simulink model "MMADC"  (R2021a)
settings: Solver=VariableStepAuto  StartTime=0.0  StopTime=1  RelTol=1e-3
values from neighbouring files (symbols this model uses):
  Cf = minimum_cap    [MMADC_main.m]
  clk_freq = 2.1*(nb_MAC+1)/nb_MAC*input_BW    (= 1684.375)    [MMADC_main.m]
  clk_period = 1/clk_freq    (= 0.000593692022263)    [MMADC_main.m]
  comparator_high_offset = 0.2*10e-4    (= 0.0002)    [MMADC_main.m]
  comparator_low_offset = -.1*10e-4    (= -0.0001)    [MMADC_main.m]
  comparator_noise_on = noise_on    (= 1)    [MMADC_main.m]
  comparator_noise_rms = 1*k*T* 2/3 / minimum_cap    [MMADC_main.m]
  comparator_offset_on = noise_on    (= 1)    [MMADC_main.m]
  k = 1.38064852e-23    [MMADC_main.m]
  LNA_bandwidth = 2.5*input_BW    (= 2000)    [MMADC_main.m]
  LNA_gain = 10^(36/20)*12*1.5849    (= 1200.00515432)    [MMADC_main.m]
  LNA_input_referred_noise = sqrt(pi/2*LNA_bandwidth*(194*10^-9)^2)    [MMADC_main.m]
  LNA_noise_on = noise_on    (= 1)    [MMADC_main.m]
  MM_incomplete_transfer_coeff = C1/(C1+C2)    [MMADC_main.m]
  MM_leakage_per_clk_cycle = 1    [MMADC_main.m]
  MM_sampling_noise = noise_on*((k*T * C1/(C1+C2)^2) + (k*T*(C1*C2/(C1+C2))/C2^2))    [MMADC_main.m]
  nb_MAC = 384    [MMADC_main.m]
  number_of_bits = 6    [MMADC_main.m]
  sample_time_jitter = 16e-12    (= 1.6e-11)    [MMADC_main.m]
  sampling_gain = Cs/Cf    [MMADC_main.m]
  sampling_jitter_on = noise_on    (= 1)    [MMADC_main.m]
  sensing_matrix = sensing_matrix_large(j:j+min(19,i-1),:)    [MMADC_main.m]
  sim_number = 0    [MMADC_main.m]
  switch_noise_on = noise_on    (= 1)    [MMADC_main.m]
  switching_noise = k*T/Cf    [MMADC_main.m]
  T = 293    [MMADC_main.m]
  Vref = 2    [MMADC_main.m]
  ZOH_delta = 0*Vref/(2^number_of_bits)    (= 0)    [MMADC_main.m]
libraries: simulink x100, simulink_extras x41, dspsigops x21, dspsrcs4 x21, spsFirstOrderFilterLib x1, dspswit3 x1
(part 2 of 10)

== system MMADC/Sensing Channel 8 ==
  In5 : Inport
  Input : Inport  Port=2
  AND : Logic  IconShape=distinctive  AllPortsSameDT=off  OutDataTypeStr=boolean
  Bus Selector : BusSelector  OutputSignals=reset MAC,trigger MAC,sample SAR,trigger SAR
  SAR : Subsystem
      mask Display: text(.5, .5, 'ZOH SAR', 'horizontalAlignment', 'center', 'verticalAlignment', 'middle')
  Sample&hold : Subsystem
      settings: PortSchema="{\"entries\":[{\"content\":{\"sides\":[{\"content\":{\"connectorIds\":[\"In1\"]},\"type\":\"ConnectorPlacement.EquallySpacedRectSide\",\"uuid\":\"7dc7a4da-613e-4b0b-8b13-7686a16d7398\"},{\"content\":{\"connectorIds\":[\"Out1\"],\"side\":\"RIGHT\"},\"type\":\"ConnectorPlacement.EquallySpacedRectSide\",\"uuid\":\"45e05abc-e512-455b-8082-6639e5b5b38c\"},{\"content\":{\"connectorIds\":[\"In2\"],\"side\":\"TOP\"},\"type\":\"ConnectorPlacement.EquallySpacedRectSide\",\"uuid\":\"b599ec83-17db-48a3-a9e2-86d99bd6436c\"},{\"content\":{\"connectorIds\":[],\"side\":\"HIDDEN\"},\"type\":\"ConnectorPlacement.EquallySpacedRectSide\",\"uuid\":\"38635b0c-9992-4d58-9e3d-95a04571faab\"}]},\"type\":\"ConnectorPlacement.EquallySpacedConnector\",\"uuid\":\"ba0d73a9-648c-4aab-96ad-c6572107f92b\"}],\"packageUris\":[\"http://schema.mathworks.com/mf0/Connector/R2020b\"],\"version\":\"1.0\"}"
      mask Display: text(.5, .5, 'Sample & hold', 'horizontalAlignment', 'center', 'verticalAlignment', 'middle')
  Signal From Workspace : dspsrcs4/Signal From Workspace  X=sensing_matrix(8,:)  Ts=clk_period  nsamps=1  OutputAfterFinalValue=Cyclic repetition  ignoreOrWarnInputAndFrameLengths=off  OutputFrames=off
  Subsystem2 : Subsystem
  " " : Outport
  wires:
  SAR/2(" ") -> " "/1
  Subsystem2/1(Out1) -> Sample&hold/1(x(t))
  In5/1 -> Subsystem2/2(In1)
  Sample&hold/1(Sampled value) -> SAR/2(Signal in)
  Input/1 -> Bus Selector/1
  Bus Selector/1 -> Subsystem2/1(Reset)  "<reset MAC>"
  Bus Selector/3 -> Sample&hold/2(Trigger)  "<sample SAR>"
  Bus Selector/4 -> SAR/1(Trigger)  "<trigger SAR>"
  AND/1 -> Subsystem2/Trigger
  Signal From Workspace/1 -> AND/2
  Bus Selector/2 -> AND/1  "<trigger MAC>"

== system MMADC/Sensing Channel 9 ==
  In5 : Inport
  Input : Inport  Port=2
  AND : Logic  IconShape=distinctive  AllPortsSameDT=off  OutDataTypeStr=boolean
  Bus Selector : BusSelector  OutputSignals=reset MAC,trigger MAC,sample SAR,trigger SAR
  SAR : Subsystem
      mask Display: text(.5, .5, 'ZOH SAR', 'horizontalAlignment', 'center', 'verticalAlignment', 'middle')
  Sample&hold : Subsystem
      settings: PortSchema="{\"entries\":[{\"content\":{\"sides\":[{\"content\":{\"connectorIds\":[\"In1\"]},\"type\":\"ConnectorPlacement.EquallySpacedRectSide\",\"uuid\":\"7dc7a4da-613e-4b0b-8b13-7686a16d7398\"},{\"content\":{\"connectorIds\":[\"Out1\"],\"side\":\"RIGHT\"},\"type\":\"ConnectorPlacement.EquallySpacedRectSide\",\"uuid\":\"45e05abc-e512-455b-8082-6639e5b5b38c\"},{\"content\":{\"connectorIds\":[\"In2\"],\"side\":\"TOP\"},\"type\":\"ConnectorPlacement.EquallySpacedRectSide\",\"uuid\":\"b599ec83-17db-48a3-a9e2-86d99bd6436c\"},{\"content\":{\"connectorIds\":[],\"side\":\"HIDDEN\"},\"type\":\"ConnectorPlacement.EquallySpacedRectSide\",\"uuid\":\"38635b0c-9992-4d58-9e3d-95a04571faab\"}]},\"type\":\"ConnectorPlacement.EquallySpacedConnector\",\"uuid\":\"ba0d73a9-648c-4aab-96ad-c6572107f92b\"}],\"packageUris\":[\"http://schema.mathworks.com/mf0/Connector/R2020b\"],\"version\":\"1.0\"}"
      mask Display: text(.5, .5, 'Sample & hold', 'horizontalAlignment', 'center', 'verticalAlignment', 'middle')
  Signal From Workspace : dspsrcs4/Signal From Workspace  X=sensing_matrix(9,:)  Ts=clk_period  nsamps=1  OutputAfterFinalValue=Cyclic repetition  ignoreOrWarnInputAndFrameLengths=off  OutputFrames=off
  Subsystem2 : Subsystem
  " " : Outport
  wires:
  SAR/2(" ") -> " "/1
  Subsystem2/1(Out1) -> Sample&hold/1(x(t))
  In5/1 -> Subsystem2/2(In1)
  Sample&hold/1(Sampled value) -> SAR/2(Signal in)
  Input/1 -> Bus Selector/1
  Bus Selector/1 -> Subsystem2/1(Reset)  "<reset MAC>"
  Bus Selector/3 -> Sample&hold/2(Trigger)  "<sample SAR>"
  Bus Selector/4 -> SAR/1(Trigger)  "<trigger SAR>"
  Signal From Workspace/1 -> AND/2
  Bus Selector/2 -> AND/1  "<trigger MAC>"
  AND/1 -> Subsystem2/Trigger

== system MMADC/Subsystem1 ==
  Input : Inport
  AND : Logic  IconShape=distinctive  AllPortsSameDT=off  OutDataTypeStr=boolean
  AND2 : Logic  IconShape=distinctive  AllPortsSameDT=off  OutDataTypeStr=boolean
  AND3 : Logic  IconShape=distinctive  AllPortsSameDT=off  OutDataTypeStr=boolean
  Bus Creator : BusCreator  Inputs=4
  Constant : Constant  Value=number_of_bits
  Constant1 : Constant  Value=nb_MAC
  Counter : dspswit3/Counter  Direction=Up  CountEvent=Rising edge  CounterSize=User defined  MaxCount=nb_MAC  InitialCount=nb_MAC  Output=Count  HitValue=32  ResetInput=on  SamplesPerFrame=1  Ts=1  CntDtype=double  HitDtype=Logical
  MATLAB Function : MATLAB Function  TreatAsAtomicUnit=on
  Output4 : Outport
  wires:
  Input/1 -> Counter/1, AND2/2, AND3/2, AND/2
  Counter/1 -> MATLAB Function/1(counter)
  Constant1/1 -> MATLAB Function/2(nb_MAC)
  AND/1 -> Bus Creator/2  "trigger MAC"
  AND2/1 -> Bus Creator/4  "trigger SAR"
  AND3/1 -> Bus Creator/3  "sample SAR"
  MATLAB Function/4(sample_SAR) -> AND3/1
  MATLAB Function/3(trigger_SAR) -> AND2/1
  MATLAB Function/2(reset_MAC) -> Bus Creator/1  "reset MAC"
  MATLAB Function/1(trigger_MAC) -> AND/1
  Bus Creator/1 -> Output4/1
  Constant/1 -> MATLAB Function/3(nb_bits)

== system MMADC/Sensing Channel 1/SAR ==
  Trigger : Inport
  Signal in : Inport  Port=2
  "           " : dspsigops/Sample and Hold  trig=Rising edge  initCond=0  latchinput=off
  Constant : Constant  Value=Vref
  Constant1 : Constant  Value=number_of_bits
  DAC : Subsystem  TreatAsAtomicUnit=on
      mask Display: text(.5, .5, 'DAC', 'horizontalAlignment', 'center', 'verticalAlignment', 'middle')
  SAR : Subsystem  TreatAsAtomicUnit=on
      mask Display: text(.5, .5, 'SAR', 'horizontalAlignment', 'center', 'verticalAlignment', 'middle')
  ZOH+comparator : Subsystem
      settings: PortSchema="{\"entries\":[{\"content\":{\"sides\":[{\"content\":{\"connectorIds\":[\"In1\",\"In2\"]},\"type\":\"ConnectorPlacement.EquallySpacedRectSide\",\"uuid\":\"7512c97b-848f-4506-b4e4-df4323ddef76\"},{\"content\":{\"connectorIds\":[\"Out1\",\"Out2\"],\"side\":\"RIGHT\"},\"type\":\"ConnectorPlacement.EquallySpacedRectSide\",\"uuid\":\"173ab639-376f-4392-8113-9f10a64ef5ba\"},{\"content\":{\"connectorIds\":[\"In3\",\"In4\"],\"side\":\"TOP\"},\"type\":\"ConnectorPlacement.EquallySpacedRectSide\",\"uuid\":\"b167df5d-9d76-4988-887c-42eca149e1c8\"},{\"content\":{\"connectorIds\":[\"Out3\"],\"side\":\"BOTTOM\"},\"type\":\"ConnectorPlacement.EquallySpacedRectSide\",\"uuid\":\"853aabd3-db33-416b-be96-d4661842c69c\"},{\"content\":{\"connectorIds\":[],\"side\":\"HIDDEN\"},\"type\":\"ConnectorPlacement.EquallySpacedRectSide\",\"uuid\":\"e2358589-1082-44c0-a092-f45782973cce\"}]},\"type\":\"ConnectorPlacement.EquallySpacedConnector\",\"uuid\":\"7d04fd09-a295-4450-8277-4727e6a38cb5\"}],\"packageUris\":[\"http://schema.mathworks.com/mf0/Connector/R2020b\"],\"version\":\"1.0\"}"
      mask Display: text(.5, .5, 'Comparator', 'horizontalAlignment', 'center', 'verticalAlignment', 'middle')
  Count ZOH's : Outport
  " " : Outport  Port=2
  wires:
  SAR/2(SAR_done) -> "           "/Trigger
  ZOH+comparator/3(Output) -> Count ZOH's/1
  SAR/3(Output_code) -> DAC/3(Input_code)
  "           "/1 -> " "/1
  Constant/1 -> DAC/2(Vref)
  ZOH+comparator/1(Output2) -> SAR/1(Comparator_in)
  Signal in/1 -> ZOH+comparator/1(Signal in)
  Constant1/1 -> SAR/3(Number of bits), DAC/1(NOB)
  DAC/1(y) -> ZOH+comparator/2(DAC in), "           "/1
  ZOH+comparator/2(Output1) -> SAR/2(ZOH)
  SAR/1(Output) -> ZOH+comparator/3(Input)
  Trigger/1 -> SAR/Trigger, ZOH+comparator/4(Clk)

== system MMADC/Sensing Channel 1/Sample&hold ==
  x(t) : Inport
  Trigger : Inport  Port=2
  Sample switch noise : Subsystem  TreatAsAtomicUnit=on
  Sample time jitter : Subsystem
  Sampled value : Outport
  wires:
  x(t)/1 -> Sample time jitter/1(x(t))
  Trigger/1 -> Sample switch noise/Trigger
  Sample switch noise/1(y(t)) -> Sampled value/1  "Sampled value"
  Sample time jitter/1(Output) -> Sample switch noise/1(Input)

== system MMADC/Sensing Channel 1/Subsystem2 ==
  Reset : Inport
  In1 : Inport  Port=2
  Trigger : TriggerPort  VariantControl=Variant  PortDimensions=1
  Add : Sum  Inputs=+++
  Constant : Constant  Value=0
  Multiply1 : Gain  Gain=MM_incomplete_transfer_coeff
  Multiply2 : Gain  Gain=MM_leakage_per_clk_cycle
  Random Number : RandomNumber  Variance=MM_sampling_noise  Seed=sim_number
  Switch : Switch  Criteria=u2 ~= 0
  Unit Delay : UnitDelay  SampleTime=-1  HasFrameUpgradeWarning=on
  Out1 : Outport
  wires:
  Add/1 -> Out1/1, Unit Delay/1  "mac out"
  Switch/1 -> Add/3  "switch out"
  In1/1 -> Multiply1/1
  Unit Delay/1 -> Multiply2/1
  Multiply2/1 -> Switch/3
  Random Number/1 -> Add/1
  Multiply1/1 -> Add/2
  Reset/1 -> Switch/2
  Constant/1 -> Switch/1

== system MMADC/Sensing Channel 10/SAR ==
  Trigger : Inport
  Signal in : Inport  Port=2
  "           " : dspsigops/Sample and Hold  trig=Rising edge  initCond=0  latchinput=off
  Constant : Constant  Value=Vref
  Constant1 : Constant  Value=number_of_bits
  DAC : Subsystem  TreatAsAtomicUnit=on
      mask Display: text(.5, .5, 'DAC', 'horizontalAlignment', 'center', 'verticalAlignment', 'middle')
  SAR : Subsystem  TreatAsAtomicUnit=on
      mask Display: text(.5, .5, 'SAR', 'horizontalAlignment', 'center', 'verticalAlignment', 'middle')
  ZOH+comparator : Subsystem
      settings: PortSchema="{\"entries\":[{\"content\":{\"sides\":[{\"content\":{\"connectorIds\":[\"In1\",\"In2\"]},\"type\":\"ConnectorPlacement.EquallySpacedRectSide\",\"uuid\":\"7512c97b-848f-4506-b4e4-df4323ddef76\"},{\"content\":{\"connectorIds\":[\"Out1\",\"Out2\"],\"side\":\"RIGHT\"},\"type\":\"ConnectorPlacement.EquallySpacedRectSide\",\"uuid\":\"173ab639-376f-4392-8113-9f10a64ef5ba\"},{\"content\":{\"connectorIds\":[\"In3\",\"In4\"],\"side\":\"TOP\"},\"type\":\"ConnectorPlacement.EquallySpacedRectSide\",\"uuid\":\"b167df5d-9d76-4988-887c-42eca149e1c8\"},{\"content\":{\"connectorIds\":[\"Out3\"],\"side\":\"BOTTOM\"},\"type\":\"ConnectorPlacement.EquallySpacedRectSide\",\"uuid\":\"853aabd3-db33-416b-be96-d4661842c69c\"},{\"content\":{\"connectorIds\":[],\"side\":\"HIDDEN\"},\"type\":\"ConnectorPlacement.EquallySpacedRectSide\",\"uuid\":\"e2358589-1082-44c0-a092-f45782973cce\"}]},\"type\":\"ConnectorPlacement.EquallySpacedConnector\",\"uuid\":\"7d04fd09-a295-4450-8277-4727e6a38cb5\"}],\"packageUris\":[\"http://schema.mathworks.com/mf0/Connector/R2020b\"],\"version\":\"1.0\"}"
      mask Display: text(.5, .5, 'Comparator', 'horizontalAlignment', 'center', 'verticalAlignment', 'middle')
  Count ZOH's : Outport
  " " : Outport  Port=2
  wires:
  SAR/2(SAR_done) -> "           "/Trigger
  ZOH+comparator/3(Output) -> Count ZOH's/1
  SAR/3(Output_code) -> DAC/3(Input_code)
  "           "/1 -> " "/1
  Constant/1 -> DAC/2(Vref)
  ZOH+comparator/1(Output2) -> SAR/1(Comparator_in)
  Signal in/1 -> ZOH+comparator/1(Signal in)
  Constant1/1 -> SAR/3(Number of bits), DAC/1(NOB)
  DAC/1(y) -> ZOH+comparator/2(DAC in), "           "/1
  ZOH+comparator/2(Output1) -> SAR/2(ZOH)
  SAR/1(Output) -> ZOH+comparator/3(Input)
  Trigger/1 -> ZOH+comparator/4(Clk), SAR/Trigger

== system MMADC/Sensing Channel 10/Sample&hold ==
  x(t) : Inport
  Trigger : Inport  Port=2
  Sample switch noise : Subsystem  TreatAsAtomicUnit=on
  Sample time jitter : Subsystem
  Sampled value : Outport
  wires:
  x(t)/1 -> Sample time jitter/1(x(t))
  Trigger/1 -> Sample switch noise/Trigger
  Sample switch noise/1(y(t)) -> Sampled value/1  "Sampled value"
  Sample time jitter/1(Output) -> Sample switch noise/1(Input)

== system MMADC/Sensing Channel 10/Subsystem2 ==
  Reset : Inport
  In1 : Inport  Port=2
  Trigger : TriggerPort  VariantControl=Variant  PortDimensions=1
  Add : Sum  Inputs=+++
  Multiply1 : Gain  Gain=MM_incomplete_transfer_coeff
  Multiply2 : Gain  Gain=MM_leakage_per_clk_cycle
  Random Number : RandomNumber  Variance=MM_sampling_noise
  Subsystem : Subsystem
  Unit Delay : UnitDelay  SampleTime=-1  HasFrameUpgradeWarning=on
  Out1 : Outport
  wires:
  Add/1 -> Out1/1, Unit Delay/1
  Reset/1 -> Subsystem/1(In1)
  Subsystem/1(Out1) -> Add/3
  In1/1 -> Multiply1/1
  Unit Delay/1 -> Multiply2/1
  Multiply2/1 -> Subsystem/2(In2)
  Random Number/1 -> Add/1
  Multiply1/1 -> Add/2

== system MMADC/Sensing Channel 11/SAR ==
  Trigger : Inport
  Signal in : Inport  Port=2
  "           " : dspsigops/Sample and Hold  trig=Rising edge  initCond=0  latchinput=off
  Constant : Constant  Value=Vref
  Constant1 : Constant  Value=number_of_bits
  DAC : Subsystem  TreatAsAtomicUnit=on
      mask Display: text(.5, .5, 'DAC', 'horizontalAlignment', 'center', 'verticalAlignment', 'middle')
  SAR : Subsystem  TreatAsAtomicUnit=on
      mask Display: text(.5, .5, 'SAR', 'horizontalAlignment', 'center', 'verticalAlignment', 'middle')
  ZOH+comparator : Subsystem
      settings: PortSchema="{\"entries\":[{\"content\":{\"sides\":[{\"content\":{\"connectorIds\":[\"In1\",\"In2\"]},\"type\":\"ConnectorPlacement.EquallySpacedRectSide\",\"uuid\":\"7512c97b-848f-4506-b4e4-df4323ddef76\"},{\"content\":{\"connectorIds\":[\"Out1\",\"Out2\"],\"side\":\"RIGHT\"},\"type\":\"ConnectorPlacement.EquallySpacedRectSide\",\"uuid\":\"173ab639-376f-4392-8113-9f10a64ef5ba\"},{\"content\":{\"connectorIds\":[\"In3\",\"In4\"],\"side\":\"TOP\"},\"type\":\"ConnectorPlacement.EquallySpacedRectSide\",\"uuid\":\"b167df5d-9d76-4988-887c-42eca149e1c8\"},{\"content\":{\"connectorIds\":[\"Out3\"],\"side\":\"BOTTOM\"},\"type\":\"ConnectorPlacement.EquallySpacedRectSide\",\"uuid\":\"853aabd3-db33-416b-be96-d4661842c69c\"},{\"content\":{\"connectorIds\":[],\"side\":\"HIDDEN\"},\"type\":\"ConnectorPlacement.EquallySpacedRectSide\",\"uuid\":\"e2358589-1082-44c0-a092-f45782973cce\"}]},\"type\":\"ConnectorPlacement.EquallySpacedConnector\",\"uuid\":\"7d04fd09-a295-4450-8277-4727e6a38cb5\"}],\"packageUris\":[\"http://schema.mathworks.com/mf0/Connector/R2020b\"],\"version\":\"1.0\"}"
      mask Display: text(.5, .5, 'Comparator', 'horizontalAlignment', 'center', 'verticalAlignment', 'middle')
  Count ZOH's : Outport
  " " : Outport  Port=2
  wires:
  SAR/2(SAR_done) -> "           "/Trigger
  ZOH+comparator/3(Output) -> Count ZOH's/1
  SAR/3(Output_code) -> DAC/3(Input_code)
  "           "/1 -> " "/1
  Constant/1 -> DAC/2(Vref)
  ZOH+comparator/1(Output2) -> SAR/1(Comparator_in)
  Signal in/1 -> ZOH+comparator/1(Signal in)
  Constant1/1 -> SAR/3(Number of bits), DAC/1(NOB)
  DAC/1(y) -> ZOH+comparator/2(DAC in), "           "/1
  ZOH+comparator/2(Output1) -> SAR/2(ZOH)
  SAR/1(Output) -> ZOH+comparator/3(Input)
  Trigger/1 -> ZOH+comparator/4(Clk), SAR/Trigger

== system MMADC/Sensing Channel 11/Sample&hold ==
  x(t) : Inport
  Trigger : Inport  Port=2
  Sample switch noise : Subsystem  TreatAsAtomicUnit=on
  Sample time jitter : Subsystem
  Sampled value : Outport
  wires:
  x(t)/1 -> Sample time jitter/1(x(t))
  Trigger/1 -> Sample switch noise/Trigger
  Sample switch noise/1(y(t)) -> Sampled value/1  "Sampled value"
  Sample time jitter/1(Output) -> Sample switch noise/1(Input)

== system MMADC/Sensing Channel 11/Subsystem2 ==
  Reset : Inport
  In1 : Inport  Port=2
  Trigger : TriggerPort  VariantControl=Variant  PortDimensions=1
  Add : Sum  Inputs=+++
  Multiply1 : Gain  Gain=MM_incomplete_transfer_coeff
  Multiply2 : Gain  Gain=MM_leakage_per_clk_cycle
  Random Number : RandomNumber  Variance=MM_sampling_noise
  Subsystem : Subsystem
  Unit Delay : UnitDelay  SampleTime=-1  HasFrameUpgradeWarning=on
  Out1 : Outport
  wires:
  Add/1 -> Out1/1, Unit Delay/1
  Reset/1 -> Subsystem/1(In1)
  Subsystem/1(Out1) -> Add/3
  In1/1 -> Multiply1/1
  Unit Delay/1 -> Multiply2/1
  Multiply2/1 -> Subsystem/2(In2)
  Random Number/1 -> Add/1
  Multiply1/1 -> Add/2

== system MMADC/Sensing Channel 12/SAR ==
  Trigger : Inport
  Signal in : Inport  Port=2
  "           " : dspsigops/Sample and Hold  trig=Rising edge  initCond=0  latchinput=off
  Constant : Constant  Value=Vref
  Constant1 : Constant  Value=number_of_bits
  DAC : Subsystem  TreatAsAtomicUnit=on
      mask Display: text(.5, .5, 'DAC', 'horizontalAlignment', 'center', 'verticalAlignment', 'middle')
  SAR : Subsystem  TreatAsAtomicUnit=on
      mask Display: text(.5, .5, 'SAR', 'horizontalAlignment', 'center', 'verticalAlignment', 'middle')
  ZOH+comparator : Subsystem
      settings: PortSchema="{\"entries\":[{\"content\":{\"sides\":[{\"content\":{\"connectorIds\":[\"In1\",\"In2\"]},\"type\":\"ConnectorPlacement.EquallySpacedRectSide\",\"uuid\":\"7512c97b-848f-4506-b4e4-df4323ddef76\"},{\"content\":{\"connectorIds\":[\"Out1\",\"Out2\"],\"side\":\"RIGHT\"},\"type\":\"ConnectorPlacement.EquallySpacedRectSide\",\"uuid\":\"173ab639-376f-4392-8113-9f10a64ef5ba\"},{\"content\":{\"connectorIds\":[\"In3\",\"In4\"],\"side\":\"TOP\"},\"type\":\"ConnectorPlacement.EquallySpacedRectSide\",\"uuid\":\"b167df5d-9d76-4988-887c-42eca149e1c8\"},{\"content\":{\"connectorIds\":[\"Out3\"],\"side\":\"BOTTOM\"},\"type\":\"ConnectorPlacement.EquallySpacedRectSide\",\"uuid\":\"853aabd3-db33-416b-be96-d4661842c69c\"},{\"content\":{\"connectorIds\":[],\"side\":\"HIDDEN\"},\"type\":\"ConnectorPlacement.EquallySpacedRectSide\",\"uuid\":\"e2358589-1082-44c0-a092-f45782973cce\"}]},\"type\":\"ConnectorPlacement.EquallySpacedConnector\",\"uuid\":\"7d04fd09-a295-4450-8277-4727e6a38cb5\"}],\"packageUris\":[\"http://schema.mathworks.com/mf0/Connector/R2020b\"],\"version\":\"1.0\"}"
      mask Display: text(.5, .5, 'Comparator', 'horizontalAlignment', 'center', 'verticalAlignment', 'middle')
  Count ZOH's : Outport
  " " : Outport  Port=2
  wires:
  SAR/2(SAR_done) -> "           "/Trigger
  ZOH+comparator/3(Output) -> Count ZOH's/1
  SAR/3(Output_code) -> DAC/3(Input_code)
  "           "/1 -> " "/1
  Constant/1 -> DAC/2(Vref)
  ZOH+comparator/1(Output2) -> SAR/1(Comparator_in)
  Signal in/1 -> ZOH+comparator/1(Signal in)
  Constant1/1 -> SAR/3(Number of bits), DAC/1(NOB)
  DAC/1(y) -> ZOH+comparator/2(DAC in), "           "/1
  ZOH+comparator/2(Output1) -> SAR/2(ZOH)
  SAR/1(Output) -> ZOH+comparator/3(Input)
  Trigger/1 -> ZOH+comparator/4(Clk), SAR/Trigger

== system MMADC/Sensing Channel 12/Sample&hold ==
  x(t) : Inport
  Trigger : Inport  Port=2
  Sample switch noise : Subsystem  TreatAsAtomicUnit=on
  Sample time jitter : Subsystem
  Sampled value : Outport
  wires:
  x(t)/1 -> Sample time jitter/1(x(t))
  Trigger/1 -> Sample switch noise/Trigger
  Sample switch noise/1(y(t)) -> Sampled value/1  "Sampled value"
  Sample time jitter/1(Output) -> Sample switch noise/1(Input)

== system MMADC/Sensing Channel 12/Subsystem2 ==
  Reset : Inport
  In1 : Inport  Port=2
  Trigger : TriggerPort  VariantControl=Variant  PortDimensions=1
  Add : Sum  Inputs=+++
  Multiply1 : Gain  Gain=MM_incomplete_transfer_coeff
  Multiply2 : Gain  Gain=MM_leakage_per_clk_cycle
  Random Number : RandomNumber  Variance=MM_sampling_noise
  Subsystem : Subsystem
  Unit Delay : UnitDelay  SampleTime=-1  HasFrameUpgradeWarning=on
  Out1 : Outport
  wires:
  Add/1 -> Out1/1, Unit Delay/1
  Reset/1 -> Subsystem/1(In1)
  Subsystem/1(Out1) -> Add/3
  In1/1 -> Multiply1/1
  Unit Delay/1 -> Multiply2/1
  Multiply2/1 -> Subsystem/2(In2)
  Random Number/1 -> Add/1
  Multiply1/1 -> Add/2

== system MMADC/Sensing Channel 13/SAR ==
  Trigger : Inport
  Signal in : Inport  Port=2
  "           " : dspsigops/Sample and Hold  trig=Rising edge  initCond=0  latchinput=off
  Constant : Constant  Value=Vref
  Constant1 : Constant  Value=number_of_bits
  DAC : Subsystem  TreatAsAtomicUnit=on
      mask Display: text(.5, .5, 'DAC', 'horizontalAlignment', 'center', 'verticalAlignment', 'middle')
  SAR : Subsystem  TreatAsAtomicUnit=on
      mask Display: text(.5, .5, 'SAR', 'horizontalAlignment', 'center', 'verticalAlignment', 'middle')
  ZOH+comparator : Subsystem
      settings: PortSchema="{\"entries\":[{\"content\":{\"sides\":[{\"content\":{\"connectorIds\":[\"In1\",\"In2\"]},\"type\":\"ConnectorPlacement.EquallySpacedRectSide\",\"uuid\":\"7512c97b-848f-4506-b4e4-df4323ddef76\"},{\"content\":{\"connectorIds\":[\"Out1\",\"Out2\"],\"side\":\"RIGHT\"},\"type\":\"ConnectorPlacement.EquallySpacedRectSide\",\"uuid\":\"173ab639-376f-4392-8113-9f10a64ef5ba\"},{\"content\":{\"connectorIds\":[\"In3\",\"In4\"],\"side\":\"TOP\"},\"type\":\"ConnectorPlacement.EquallySpacedRectSide\",\"uuid\":\"b167df5d-9d76-4988-887c-42eca149e1c8\"},{\"content\":{\"connectorIds\":[\"Out3\"],\"side\":\"BOTTOM\"},\"type\":\"ConnectorPlacement.EquallySpacedRectSide\",\"uuid\":\"853aabd3-db33-416b-be96-d4661842c69c\"},{\"content\":{\"connectorIds\":[],\"side\":\"HIDDEN\"},\"type\":\"ConnectorPlacement.EquallySpacedRectSide\",\"uuid\":\"e2358589-1082-44c0-a092-f45782973cce\"}]},\"type\":\"ConnectorPlacement.EquallySpacedConnector\",\"uuid\":\"7d04fd09-a295-4450-8277-4727e6a38cb5\"}],\"packageUris\":[\"http://schema.mathworks.com/mf0/Connector/R2020b\"],\"version\":\"1.0\"}"
      mask Display: text(.5, .5, 'Comparator', 'horizontalAlignment', 'center', 'verticalAlignment', 'middle')
  Count ZOH's : Outport
  " " : Outport  Port=2
  wires:
  SAR/2(SAR_done) -> "           "/Trigger
  ZOH+comparator/3(Output) -> Count ZOH's/1
  SAR/3(Output_code) -> DAC/3(Input_code)
  "           "/1 -> " "/1
  Constant/1 -> DAC/2(Vref)
  ZOH+comparator/1(Output2) -> SAR/1(Comparator_in)
  Signal in/1 -> ZOH+comparator/1(Signal in)
  Constant1/1 -> SAR/3(Number of bits), DAC/1(NOB)
  DAC/1(y) -> ZOH+comparator/2(DAC in), "           "/1
  ZOH+comparator/2(Output1) -> SAR/2(ZOH)
  SAR/1(Output) -> ZOH+comparator/3(Input)
  Trigger/1 -> ZOH+comparator/4(Clk), SAR/Trigger

== system MMADC/Sensing Channel 13/Sample&hold ==
  x(t) : Inport
  Trigger : Inport  Port=2
  Sample switch noise : Subsystem  TreatAsAtomicUnit=on
  Sample time jitter : Subsystem
  Sampled value : Outport
  wires:
  x(t)/1 -> Sample time jitter/1(x(t))
  Trigger/1 -> Sample switch noise/Trigger
  Sample switch noise/1(y(t)) -> Sampled value/1  "Sampled value"
  Sample time jitter/1(Output) -> Sample switch noise/1(Input)

== system MMADC/Sensing Channel 13/Subsystem2 ==
  Reset : Inport
  In1 : Inport  Port=2
  Trigger : TriggerPort  VariantControl=Variant  PortDimensions=1
  Add : Sum  Inputs=+++
  Multiply1 : Gain  Gain=MM_incomplete_transfer_coeff
  Multiply2 : Gain  Gain=MM_leakage_per_clk_cycle
  Random Number : RandomNumber  Variance=MM_sampling_noise
  Subsystem : Subsystem
  Unit Delay : UnitDelay  SampleTime=-1  HasFrameUpgradeWarning=on
  Out1 : Outport
  wires:
  Add/1 -> Out1/1, Unit Delay/1
  Reset/1 -> Subsystem/1(In1)
  Subsystem/1(Out1) -> Add/3
  In1/1 -> Multiply1/1
  Unit Delay/1 -> Multiply2/1
  Multiply2/1 -> Subsystem/2(In2)
  Random Number/1 -> Add/1
  Multiply1/1 -> Add/2

== system MMADC/Sensing Channel 14/SAR ==
  Trigger : Inport
  Signal in : Inport  Port=2
  "           " : dspsigops/Sample and Hold  trig=Rising edge  initCond=0  latchinput=off
  Constant : Constant  Value=Vref
  Constant1 : Constant  Value=number_of_bits
  DAC : Subsystem  TreatAsAtomicUnit=on
      mask Display: text(.5, .5, 'DAC', 'horizontalAlignment', 'center', 'verticalAlignment', 'middle')
  SAR : Subsystem  TreatAsAtomicUnit=on
      mask Display: text(.5, .5, 'SAR', 'horizontalAlignment', 'center', 'verticalAlignment', 'middle')
  ZOH+comparator : Subsystem
      settings: PortSchema="{\"entries\":[{\"content\":{\"sides\":[{\"content\":{\"connectorIds\":[\"In1\",\"In2\"]},\"type\":\"ConnectorPlacement.EquallySpacedRectSide\",\"uuid\":\"7512c97b-848f-4506-b4e4-df4323ddef76\"},{\"content\":{\"connectorIds\":[\"Out1\",\"Out2\"],\"side\":\"RIGHT\"},\"type\":\"ConnectorPlacement.EquallySpacedRectSide\",\"uuid\":\"173ab639-376f-4392-8113-9f10a64ef5ba\"},{\"content\":{\"connectorIds\":[\"In3\",\"In4\"],\"side\":\"TOP\"},\"type\":\"ConnectorPlacement.EquallySpacedRectSide\",\"uuid\":\"b167df5d-9d76-4988-887c-42eca149e1c8\"},{\"content\":{\"connectorIds\":[\"Out3\"],\"side\":\"BOTTOM\"},\"type\":\"ConnectorPlacement.EquallySpacedRectSide\",\"uuid\":\"853aabd3-db33-416b-be96-d4661842c69c\"},{\"content\":{\"connectorIds\":[],\"side\":\"HIDDEN\"},\"type\":\"ConnectorPlacement.EquallySpacedRectSide\",\"uuid\":\"e2358589-1082-44c0-a092-f45782973cce\"}]},\"type\":\"ConnectorPlacement.EquallySpacedConnector\",\"uuid\":\"7d04fd09-a295-4450-8277-4727e6a38cb5\"}],\"packageUris\":[\"http://schema.mathworks.com/mf0/Connector/R2020b\"],\"version\":\"1.0\"}"
      mask Display: text(.5, .5, 'Comparator', 'horizontalAlignment', 'center', 'verticalAlignment', 'middle')
  Count ZOH's : Outport
  " " : Outport  Port=2
  wires:
  SAR/2(SAR_done) -> "           "/Trigger
  ZOH+comparator/3(Output) -> Count ZOH's/1
  SAR/3(Output_code) -> DAC/3(Input_code)
  "           "/1 -> " "/1
  Constant/1 -> DAC/2(Vref)
  ZOH+comparator/1(Output2) -> SAR/1(Comparator_in)
  Signal in/1 -> ZOH+comparator/1(Signal in)
  Constant1/1 -> SAR/3(Number of bits), DAC/1(NOB)
  DAC/1(y) -> ZOH+comparator/2(DAC in), "           "/1
  ZOH+comparator/2(Output1) -> SAR/2(ZOH)
  SAR/1(Output) -> ZOH+comparator/3(Input)
  Trigger/1 -> ZOH+comparator/4(Clk), SAR/Trigger

== system MMADC/Sensing Channel 14/Sample&hold ==
  x(t) : Inport
  Trigger : Inport  Port=2
  Sample switch noise : Subsystem  TreatAsAtomicUnit=on
  Sample time jitter : Subsystem
  Sampled value : Outport
  wires:
  x(t)/1 -> Sample time jitter/1(x(t))
  Trigger/1 -> Sample switch noise/Trigger
  Sample switch noise/1(y(t)) -> Sampled value/1  "Sampled value"
  Sample time jitter/1(Output) -> Sample switch noise/1(Input)

== system MMADC/Sensing Channel 14/Subsystem2 ==
  Reset : Inport
  In1 : Inport  Port=2
  Trigger : TriggerPort  VariantControl=Variant  PortDimensions=1
  Add : Sum  Inputs=+++
  Multiply1 : Gain  Gain=MM_incomplete_transfer_coeff
  Multiply2 : Gain  Gain=MM_leakage_per_clk_cycle
  Random Number : RandomNumber  Variance=MM_sampling_noise
  Subsystem : Subsystem
  Unit Delay : UnitDelay  SampleTime=-1  HasFrameUpgradeWarning=on
  Out1 : Outport
  wires:
  Add/1 -> Out1/1, Unit Delay/1
  Reset/1 -> Subsystem/1(In1)
  Subsystem/1(Out1) -> Add/3
  In1/1 -> Multiply1/1
  Unit Delay/1 -> Multiply2/1
  Multiply2/1 -> Subsystem/2(In2)
  Random Number/1 -> Add/1
  Multiply1/1 -> Add/2

== system MMADC/Sensing Channel 15/SAR ==
  Trigger : Inport
  Signal in : Inport  Port=2
  "           " : dspsigops/Sample and Hold  trig=Rising edge  initCond=0  latchinput=off
  Constant : Constant  Value=Vref
  Constant1 : Constant  Value=number_of_bits
  DAC : Subsystem  TreatAsAtomicUnit=on
      mask Display: text(.5, .5, 'DAC', 'horizontalAlignment', 'center', 'verticalAlignment', 'middle')
  SAR : Subsystem  TreatAsAtomicUnit=on
      mask Display: text(.5, .5, 'SAR', 'horizontalAlignment', 'center', 'verticalAlignment', 'middle')
  ZOH+comparator : Subsystem
      settings: PortSchema="{\"entries\":[{\"content\":{\"sides\":[{\"content\":{\"connectorIds\":[\"In1\",\"In2\"]},\"type\":\"ConnectorPlacement.EquallySpacedRectSide\",\"uuid\":\"7512c97b-848f-4506-b4e4-df4323ddef76\"},{\"content\":{\"connectorIds\":[\"Out1\",\"Out2\"],\"side\":\"RIGHT\"},\"type\":\"ConnectorPlacement.EquallySpacedRectSide\",\"uuid\":\"173ab639-376f-4392-8113-9f10a64ef5ba\"},{\"content\":{\"connectorIds\":[\"In3\",\"In4\"],\"side\":\"TOP\"},\"type\":\"ConnectorPlacement.EquallySpacedRectSide\",\"uuid\":\"b167df5d-9d76-4988-887c-42eca149e1c8\"},{\"content\":{\"connectorIds\":[\"Out3\"],\"side\":\"BOTTOM\"},\"type\":\"ConnectorPlacement.EquallySpacedRectSide\",\"uuid\":\"853aabd3-db33-416b-be96-d4661842c69c\"},{\"content\":{\"connectorIds\":[],\"side\":\"HIDDEN\"},\"type\":\"ConnectorPlacement.EquallySpacedRectSide\",\"uuid\":\"e2358589-1082-44c0-a092-f45782973cce\"}]},\"type\":\"ConnectorPlacement.EquallySpacedConnector\",\"uuid\":\"7d04fd09-a295-4450-8277-4727e6a38cb5\"}],\"packageUris\":[\"http://schema.mathworks.com/mf0/Connector/R2020b\"],\"version\":\"1.0\"}"
      mask Display: text(.5, .5, 'Comparator', 'horizontalAlignment', 'center', 'verticalAlignment', 'middle')
  Count ZOH's : Outport
  " " : Outport  Port=2
  wires:
  SAR/2(SAR_done) -> "           "/Trigger
  ZOH+comparator/3(Output) -> Count ZOH's/1
  SAR/3(Output_code) -> DAC/3(Input_code)
  "           "/1 -> " "/1
  Constant/1 -> DAC/2(Vref)
  ZOH+comparator/1(Output2) -> SAR/1(Comparator_in)
  Signal in/1 -> ZOH+comparator/1(Signal in)
  Constant1/1 -> SAR/3(Number of bits), DAC/1(NOB)
  DAC/1(y) -> ZOH+comparator/2(DAC in), "           "/1
  ZOH+comparator/2(Output1) -> SAR/2(ZOH)
  SAR/1(Output) -> ZOH+comparator/3(Input)
  Trigger/1 -> ZOH+comparator/4(Clk), SAR/Trigger

== system MMADC/Sensing Channel 15/Sample&hold ==
  x(t) : Inport
  Trigger : Inport  Port=2
  Sample switch noise : Subsystem  TreatAsAtomicUnit=on
  Sample time jitter : Subsystem
  Sampled value : Outport
  wires:
  x(t)/1 -> Sample time jitter/1(x(t))
  Trigger/1 -> Sample switch noise/Trigger
  Sample switch noise/1(y(t)) -> Sampled value/1  "Sampled value"
  Sample time jitter/1(Output) -> Sample switch noise/1(Input)

== system MMADC/Sensing Channel 15/Subsystem2 ==
  Reset : Inport
  In1 : Inport  Port=2
  Trigger : TriggerPort  VariantControl=Variant  PortDimensions=1
  Add : Sum  Inputs=+++
  Multiply1 : Gain  Gain=MM_incomplete_transfer_coeff
  Multiply2 : Gain  Gain=MM_leakage_per_clk_cycle
  Random Number : RandomNumber  Variance=MM_sampling_noise
  Subsystem : Subsystem
  Unit Delay : UnitDelay  SampleTime=-1  HasFrameUpgradeWarning=on
  Out1 : Outport
  wires:
  Add/1 -> Out1/1, Unit Delay/1
  Reset/1 -> Subsystem/1(In1)
  Subsystem/1(Out1) -> Add/3
  In1/1 -> Multiply1/1
  Unit Delay/1 -> Multiply2/1
  Multiply2/1 -> Subsystem/2(In2)
  Random Number/1 -> Add/1
  Multiply1/1 -> Add/2

== system MMADC/Sensing Channel 16/SAR ==
  Trigger : Inport
  Signal in : Inport  Port=2
  "           " : dspsigops/Sample and Hold  trig=Rising edge  initCond=0  latchinput=off
  Constant : Constant  Value=Vref
  Constant1 : Constant  Value=number_of_bits
  DAC : Subsystem  TreatAsAtomicUnit=on
      mask Display: text(.5, .5, 'DAC', 'horizontalAlignment', 'center', 'verticalAlignment', 'middle')
  SAR : Subsystem  TreatAsAtomicUnit=on
      mask Display: text(.5, .5, 'SAR', 'horizontalAlignment', 'center', 'verticalAlignment', 'middle')
  ZOH+comparator : Subsystem
      settings: PortSchema="{\"entries\":[{\"content\":{\"sides\":[{\"content\":{\"connectorIds\":[\"In1\",\"In2\"]},\"type\":\"ConnectorPlacement.EquallySpacedRectSide\",\"uuid\":\"7512c97b-848f-4506-b4e4-df4323ddef76\"},{\"content\":{\"connectorIds\":[\"Out1\",\"Out2\"],\"side\":\"RIGHT\"},\"type\":\"ConnectorPlacement.EquallySpacedRectSide\",\"uuid\":\"173ab639-376f-4392-8113-9f10a64ef5ba\"},{\"content\":{\"connectorIds\":[\"In3\",\"In4\"],\"side\":\"TOP\"},\"type\":\"ConnectorPlacement.EquallySpacedRectSide\",\"uuid\":\"b167df5d-9d76-4988-887c-42eca149e1c8\"},{\"content\":{\"connectorIds\":[\"Out3\"],\"side\":\"BOTTOM\"},\"type\":\"ConnectorPlacement.EquallySpacedRectSide\",\"uuid\":\"853aabd3-db33-416b-be96-d4661842c69c\"},{\"content\":{\"connectorIds\":[],\"side\":\"HIDDEN\"},\"type\":\"ConnectorPlacement.EquallySpacedRectSide\",\"uuid\":\"e2358589-1082-44c0-a092-f45782973cce\"}]},\"type\":\"ConnectorPlacement.EquallySpacedConnector\",\"uuid\":\"7d04fd09-a295-4450-8277-4727e6a38cb5\"}],\"packageUris\":[\"http://schema.mathworks.com/mf0/Connector/R2020b\"],\"version\":\"1.0\"}"
      mask Display: text(.5, .5, 'Comparator', 'horizontalAlignment', 'center', 'verticalAlignment', 'middle')
  Count ZOH's : Outport
  " " : Outport  Port=2
  wires:
  SAR/2(SAR_done) -> "           "/Trigger
  ZOH+comparator/3(Output) -> Count ZOH's/1
  SAR/3(Output_code) -> DAC/3(Input_code)
  "           "/1 -> " "/1
  Constant/1 -> DAC/2(Vref)
  ZOH+comparator/1(Output2) -> SAR/1(Comparator_in)
  Signal in/1 -> ZOH+comparator/1(Signal in)
  Constant1/1 -> SAR/3(Number of bits), DAC/1(NOB)
  DAC/1(y) -> ZOH+comparator/2(DAC in), "           "/1
  ZOH+comparator/2(Output1) -> SAR/2(ZOH)
  SAR/1(Output) -> ZOH+comparator/3(Input)
  Trigger/1 -> ZOH+comparator/4(Clk), SAR/Trigger

== system MMADC/Sensing Channel 16/Sample&hold ==
  x(t) : Inport
  Trigger : Inport  Port=2
  Sample switch noise : Subsystem  TreatAsAtomicUnit=on
  Sample time jitter : Subsystem
  Sampled value : Outport
  wires:
  x(t)/1 -> Sample time jitter/1(x(t))
  Trigger/1 -> Sample switch noise/Trigger
  Sample switch noise/1(y(t)) -> Sampled value/1  "Sampled value"
  Sample time jitter/1(Output) -> Sample switch noise/1(Input)

== system MMADC/Sensing Channel 16/Subsystem2 ==
  Reset : Inport
  In1 : Inport  Port=2
  Trigger : TriggerPort  VariantControl=Variant  PortDimensions=1
  Add : Sum  Inputs=+++
  Multiply1 : Gain  Gain=MM_incomplete_transfer_coeff
  Multiply2 : Gain  Gain=MM_leakage_per_clk_cycle
  Random Number : RandomNumber  Variance=MM_sampling_noise
  Subsystem : Subsystem
  Unit Delay : UnitDelay  SampleTime=-1  HasFrameUpgradeWarning=on
  Out1 : Outport
  wires:
  Add/1 -> Out1/1, Unit Delay/1
  Reset/1 -> Subsystem/1(In1)
  Subsystem/1(Out1) -> Add/3
  In1/1 -> Multiply1/1
  Unit Delay/1 -> Multiply2/1
  Multiply2/1 -> Subsystem/2(In2)
  Random Number/1 -> Add/1
  Multiply1/1 -> Add/2

== system MMADC/Sensing Channel 17/SAR ==
  Trigger : Inport
  Signal in : Inport  Port=2
  "           " : dspsigops/Sample and Hold  trig=Rising edge  initCond=0  latchinput=off
  Constant : Constant  Value=Vref
  Constant1 : Constant  Value=number_of_bits
  DAC : Subsystem  TreatAsAtomicUnit=on
      mask Display: text(.5, .5, 'DAC', 'horizontalAlignment', 'center', 'verticalAlignment', 'middle')
  SAR : Subsystem  TreatAsAtomicUnit=on
      mask Display: text(.5, .5, 'SAR', 'horizontalAlignment', 'center', 'verticalAlignment', 'middle')
  ZOH+comparator : Subsystem
      settings: PortSchema="{\"entries\":[{\"content\":{\"sides\":[{\"content\":{\"connectorIds\":[\"In1\",\"In2\"]},\"type\":\"ConnectorPlacement.EquallySpacedRectSide\",\"uuid\":\"7512c97b-848f-4506-b4e4-df4323ddef76\"},{\"content\":{\"connectorIds\":[\"Out1\",\"Out2\"],\"side\":\"RIGHT\"},\"type\":\"ConnectorPlacement.EquallySpacedRectSide\",\"uuid\":\"173ab639-376f-4392-8113-9f10a64ef5ba\"},{\"content\":{\"connectorIds\":[\"In3\",\"In4\"],\"side\":\"TOP\"},\"type\":\"ConnectorPlacement.EquallySpacedRectSide\",\"uuid\":\"b167df5d-9d76-4988-887c-42eca149e1c8\"},{\"content\":{\"connectorIds\":[\"Out3\"],\"side\":\"BOTTOM\"},\"type\":\"ConnectorPlacement.EquallySpacedRectSide\",\"uuid\":\"853aabd3-db33-416b-be96-d4661842c69c\"},{\"content\":{\"connectorIds\":[],\"side\":\"HIDDEN\"},\"type\":\"ConnectorPlacement.EquallySpacedRectSide\",\"uuid\":\"e2358589-1082-44c0-a092-f45782973cce\"}]},\"type\":\"ConnectorPlacement.EquallySpacedConnector\",\"uuid\":\"7d04fd09-a295-4450-8277-4727e6a38cb5\"}],\"packageUris\":[\"http://schema.mathworks.com/mf0/Connector/R2020b\"],\"version\":\"1.0\"}"
      mask Display: text(.5, .5, 'Comparator', 'horizontalAlignment', 'center', 'verticalAlignment', 'middle')
  Count ZOH's : Outport
  " " : Outport  Port=2
  wires:
  SAR/2(SAR_done) -> "           "/Trigger
  ZOH+comparator/3(Output) -> Count ZOH's/1
  SAR/3(Output_code) -> DAC/3(Input_code)
  "           "/1 -> " "/1
  Constant/1 -> DAC/2(Vref)
  ZOH+comparator/1(Output2) -> SAR/1(Comparator_in)
  Signal in/1 -> ZOH+comparator/1(Signal in)
  Constant1/1 -> SAR/3(Number of bits), DAC/1(NOB)
  DAC/1(y) -> ZOH+comparator/2(DAC in), "           "/1
  ZOH+comparator/2(Output1) -> SAR/2(ZOH)
  SAR/1(Output) -> ZOH+comparator/3(Input)
  Trigger/1 -> ZOH+comparator/4(Clk), SAR/Trigger

== system MMADC/Sensing Channel 17/Sample&hold ==
  x(t) : Inport
  Trigger : Inport  Port=2
  Sample switch noise : Subsystem  TreatAsAtomicUnit=on
  Sample time jitter : Subsystem
  Sampled value : Outport
  wires:
  x(t)/1 -> Sample time jitter/1(x(t))
  Trigger/1 -> Sample switch noise/Trigger
  Sample switch noise/1(y(t)) -> Sampled value/1  "Sampled value"
  Sample time jitter/1(Output) -> Sample switch noise/1(Input)

== system MMADC/Sensing Channel 17/Subsystem2 ==
  Reset : Inport
  In1 : Inport  Port=2
  Trigger : TriggerPort  VariantControl=Variant  PortDimensions=1
  Add : Sum  Inputs=+++
  Multiply1 : Gain  Gain=MM_incomplete_transfer_coeff
  Multiply2 : Gain  Gain=MM_leakage_per_clk_cycle
  Random Number : RandomNumber  Variance=MM_sampling_noise
  Subsystem : Subsystem
  Unit Delay : UnitDelay  SampleTime=-1  HasFrameUpgradeWarning=on
  Out1 : Outport
  wires:
  Add/1 -> Out1/1, Unit Delay/1
  Reset/1 -> Subsystem/1(In1)
  Subsystem/1(Out1) -> Add/3
  In1/1 -> Multiply1/1
  Unit Delay/1 -> Multiply2/1
  Multiply2/1 -> Subsystem/2(In2)
  Random Number/1 -> Add/1
  Multiply1/1 -> Add/2

== system MMADC/Sensing Channel 18/SAR ==
  Trigger : Inport
  Signal in : Inport  Port=2
  "           " : dspsigops/Sample and Hold  trig=Rising edge  initCond=0  latchinput=off
  Constant : Constant  Value=Vref
  Constant1 : Constant  Value=number_of_bits
  DAC : Subsystem  TreatAsAtomicUnit=on
      mask Display: text(.5, .5, 'DAC', 'horizontalAlignment', 'center', 'verticalAlignment', 'middle')
  SAR : Subsystem  TreatAsAtomicUnit=on
      mask Display: text(.5, .5, 'SAR', 'horizontalAlignment', 'center', 'verticalAlignment', 'middle')
  ZOH+comparator : Subsystem
      settings: PortSchema="{\"entries\":[{\"content\":{\"sides\":[{\"content\":{\"connectorIds\":[\"In1\",\"In2\"]},\"type\":\"ConnectorPlacement.EquallySpacedRectSide\",\"uuid\":\"7512c97b-848f-4506-b4e4-df4323ddef76\"},{\"content\":{\"connectorIds\":[\"Out1\",\"Out2\"],\"side\":\"RIGHT\"},\"type\":\"ConnectorPlacement.EquallySpacedRectSide\",\"uuid\":\"173ab639-376f-4392-8113-9f10a64ef5ba\"},{\"content\":{\"connectorIds\":[\"In3\",\"In4\"],\"side\":\"TOP\"},\"type\":\"ConnectorPlacement.EquallySpacedRectSide\",\"uuid\":\"b167df5d-9d76-4988-887c-42eca149e1c8\"},{\"content\":{\"connectorIds\":[\"Out3\"],\"side\":\"BOTTOM\"},\"type\":\"ConnectorPlacement.EquallySpacedRectSide\",\"uuid\":\"853aabd3-db33-416b-be96-d4661842c69c\"},{\"content\":{\"connectorIds\":[],\"side\":\"HIDDEN\"},\"type\":\"ConnectorPlacement.EquallySpacedRectSide\",\"uuid\":\"e2358589-1082-44c0-a092-f45782973cce\"}]},\"type\":\"ConnectorPlacement.EquallySpacedConnector\",\"uuid\":\"7d04fd09-a295-4450-8277-4727e6a38cb5\"}],\"packageUris\":[\"http://schema.mathworks.com/mf0/Connector/R2020b\"],\"version\":\"1.0\"}"
      mask Display: text(.5, .5, 'Comparator', 'horizontalAlignment', 'center', 'verticalAlignment', 'middle')
  Count ZOH's : Outport
  " " : Outport  Port=2
  wires:
  SAR/2(SAR_done) -> "           "/Trigger
  ZOH+comparator/3(Output) -> Count ZOH's/1
  SAR/3(Output_code) -> DAC/3(Input_code)
  "           "/1 -> " "/1
  Constant/1 -> DAC/2(Vref)
  ZOH+comparator/1(Output2) -> SAR/1(Comparator_in)
  Signal in/1 -> ZOH+comparator/1(Signal in)
  Constant1/1 -> SAR/3(Number of bits), DAC/1(NOB)
  DAC/1(y) -> ZOH+comparator/2(DAC in), "           "/1
  ZOH+comparator/2(Output1) -> SAR/2(ZOH)
  SAR/1(Output) -> ZOH+comparator/3(Input)
  Trigger/1 -> ZOH+comparator/4(Clk), SAR/Trigger

== system MMADC/Sensing Channel 18/Sample&hold ==
  x(t) : Inport
  Trigger : Inport  Port=2
  Sample switch noise : Subsystem  TreatAsAtomicUnit=on
  Sample time jitter : Subsystem
  Sampled value : Outport
  wires:
  x(t)/1 -> Sample time jitter/1(x(t))
  Trigger/1 -> Sample switch noise/Trigger
  Sample switch noise/1(y(t)) -> Sampled value/1  "Sampled value"
  Sample time jitter/1(Output) -> Sample switch noise/1(Input)

== system MMADC/Sensing Channel 18/Subsystem2 ==
  Reset : Inport
  In1 : Inport  Port=2
  Trigger : TriggerPort  VariantControl=Variant  PortDimensions=1
  Add : Sum  Inputs=+++
  Multiply1 : Gain  Gain=MM_incomplete_transfer_coeff
  Multiply2 : Gain  Gain=MM_leakage_per_clk_cycle
  Random Number : RandomNumber  Variance=MM_sampling_noise
  Subsystem : Subsystem
  Unit Delay : UnitDelay  SampleTime=-1  HasFrameUpgradeWarning=on
  Out1 : Outport
  wires:
  Add/1 -> Out1/1, Unit Delay/1
  Reset/1 -> Subsystem/1(In1)
  Subsystem/1(Out1) -> Add/3
  In1/1 -> Multiply1/1
  Unit Delay/1 -> Multiply2/1
  Multiply2/1 -> Subsystem/2(In2)
  Random Number/1 -> Add/1
  Multiply1/1 -> Add/2

== system MMADC/Sensing Channel 19/SAR ==
  Trigger : Inport
  Signal in : Inport  Port=2
  "           " : dspsigops/Sample and Hold  trig=Rising edge  initCond=0  latchinput=off
  Constant : Constant  Value=Vref
  Constant1 : Constant  Value=number_of_bits
  DAC : Subsystem  TreatAsAtomicUnit=on
      mask Display: text(.5, .5, 'DAC', 'horizontalAlignment', 'center', 'verticalAlignment', 'middle')
  SAR : Subsystem  TreatAsAtomicUnit=on
      mask Display: text(.5, .5, 'SAR', 'horizontalAlignment', 'center', 'verticalAlignment', 'middle')
  ZOH+comparator : Subsystem
      settings: PortSchema="{\"entries\":[{\"content\":{\"sides\":[{\"content\":{\"connectorIds\":[\"In1\",\"In2\"]},\"type\":\"ConnectorPlacement.EquallySpacedRectSide\",\"uuid\":\"7512c97b-848f-4506-b4e4-df4323ddef76\"},{\"content\":{\"connectorIds\":[\"Out1\",\"Out2\"],\"side\":\"RIGHT\"},\"type\":\"ConnectorPlacement.EquallySpacedRectSide\",\"uuid\":\"173ab639-376f-4392-8113-9f10a64ef5ba\"},{\"content\":{\"connectorIds\":[\"In3\",\"In4\"],\"side\":\"TOP\"},\"type\":\"ConnectorPlacement.EquallySpacedRectSide\",\"uuid\":\"b167df5d-9d76-4988-887c-42eca149e1c8\"},{\"content\":{\"connectorIds\":[\"Out3\"],\"side\":\"BOTTOM\"},\"type\":\"ConnectorPlacement.EquallySpacedRectSide\",\"uuid\":\"853aabd3-db33-416b-be96-d4661842c69c\"},{\"content\":{\"connectorIds\":[],\"side\":\"HIDDEN\"},\"type\":\"ConnectorPlacement.EquallySpacedRectSide\",\"uuid\":\"e2358589-1082-44c0-a092-f45782973cce\"}]},\"type\":\"ConnectorPlacement.EquallySpacedConnector\",\"uuid\":\"7d04fd09-a295-4450-8277-4727e6a38cb5\"}],\"packageUris\":[\"http://schema.mathworks.com/mf0/Connector/R2020b\"],\"version\":\"1.0\"}"
      mask Display: text(.5, .5, 'Comparator', 'horizontalAlignment', 'center', 'verticalAlignment', 'middle')
  Count ZOH's : Outport
  " " : Outport  Port=2
  wires:
  SAR/2(SAR_done) -> "           "/Trigger
  ZOH+comparator/3(Output) -> Count ZOH's/1
  SAR/3(Output_code) -> DAC/3(Input_code)
  "           "/1 -> " "/1
  Constant/1 -> DAC/2(Vref)
  ZOH+comparator/1(Output2) -> SAR/1(Comparator_in)
  Signal in/1 -> ZOH+comparator/1(Signal in)
  Constant1/1 -> SAR/3(Number of bits), DAC/1(NOB)
  DAC/1(y) -> ZOH+comparator/2(DAC in), "           "/1
  ZOH+comparator/2(Output1) -> SAR/2(ZOH)
  SAR/1(Output) -> ZOH+comparator/3(Input)
  Trigger/1 -> ZOH+comparator/4(Clk), SAR/Trigger

== system MMADC/Sensing Channel 19/Sample&hold ==
  x(t) : Inport
  Trigger : Inport  Port=2
  Sample switch noise : Subsystem  TreatAsAtomicUnit=on
  Sample time jitter : Subsystem
  Sampled value : Outport
  wires:
  x(t)/1 -> Sample time jitter/1(x(t))
  Trigger/1 -> Sample switch noise/Trigger
  Sample switch noise/1(y(t)) -> Sampled value/1  "Sampled value"
  Sample time jitter/1(Output) -> Sample switch noise/1(Input)

== system MMADC/Sensing Channel 19/Subsystem2 ==
  Reset : Inport
  In1 : Inport  Port=2
  Trigger : TriggerPort  VariantControl=Variant  PortDimensions=1
  Add : Sum  Inputs=+++
  Multiply1 : Gain  Gain=MM_incomplete_transfer_coeff
  Multiply2 : Gain  Gain=MM_leakage_per_clk_cycle
  Random Number : RandomNumber  Variance=MM_sampling_noise
  Subsystem : Subsystem
  Unit Delay : UnitDelay  SampleTime=-1  HasFrameUpgradeWarning=on
  Out1 : Outport
  wires:
  Add/1 -> Out1/1, Unit Delay/1
  Reset/1 -> Subsystem/1(In1)
  Subsystem/1(Out1) -> Add/3
  In1/1 -> Multiply1/1
  Unit Delay/1 -> Multiply2/1
  Multiply2/1 -> Subsystem/2(In2)
  Random Number/1 -> Add/1
  Multiply1/1 -> Add/2

== system MMADC/Sensing Channel 2/SAR ==
  Trigger : Inport
  Signal in : Inport  Port=2
  "           " : dspsigops/Sample and Hold  trig=Rising edge  initCond=0  latchinput=off
  Constant : Constant  Value=Vref
  Constant1 : Constant  Value=number_of_bits
  DAC : Subsystem  TreatAsAtomicUnit=on
      mask Display: text(.5, .5, 'DAC', 'horizontalAlignment', 'center', 'verticalAlignment', 'middle')
  SAR : Subsystem  TreatAsAtomicUnit=on
      mask Display: text(.5, .5, 'SAR', 'horizontalAlignment', 'center', 'verticalAlignment', 'middle')
  ZOH+comparator : Subsystem
      settings: PortSchema="{\"entries\":[{\"content\":{\"sides\":[{\"content\":{\"connectorIds\":[\"In1\",\"In2\"]},\"type\":\"ConnectorPlacement.EquallySpacedRectSide\",\"uuid\":\"7512c97b-848f-4506-b4e4-df4323ddef76\"},{\"content\":{\"connectorIds\":[\"Out1\",\"Out2\"],\"side\":\"RIGHT\"},\"type\":\"ConnectorPlacement.EquallySpacedRectSide\",\"uuid\":\"173ab639-376f-4392-8113-9f10a64ef5ba\"},{\"content\":{\"connectorIds\":[\"In3\",\"In4\"],\"side\":\"TOP\"},\"type\":\"ConnectorPlacement.EquallySpacedRectSide\",\"uuid\":\"b167df5d-9d76-4988-887c-42eca149e1c8\"},{\"content\":{\"connectorIds\":[\"Out3\"],\"side\":\"BOTTOM\"},\"type\":\"ConnectorPlacement.EquallySpacedRectSide\",\"uuid\":\"853aabd3-db33-416b-be96-d4661842c69c\"},{\"content\":{\"connectorIds\":[],\"side\":\"HIDDEN\"},\"type\":\"ConnectorPlacement.EquallySpacedRectSide\",\"uuid\":\"e2358589-1082-44c0-a092-f45782973cce\"}]},\"type\":\"ConnectorPlacement.EquallySpacedConnector\",\"uuid\":\"7d04fd09-a295-4450-8277-4727e6a38cb5\"}],\"packageUris\":[\"http://schema.mathworks.com/mf0/Connector/R2020b\"],\"version\":\"1.0\"}"
      mask Display: text(.5, .5, 'Comparator', 'horizontalAlignment', 'center', 'verticalAlignment', 'middle')
  Count ZOH's : Outport
  " " : Outport  Port=2
  wires:
  SAR/2(SAR_done) -> "           "/Trigger
  ZOH+comparator/3(Output) -> Count ZOH's/1
  SAR/3(Output_code) -> DAC/3(Input_code)
  "           "/1 -> " "/1
  Constant/1 -> DAC/2(Vref)
  ZOH+comparator/1(Output2) -> SAR/1(Comparator_in)
  Signal in/1 -> ZOH+comparator/1(Signal in)
  Constant1/1 -> SAR/3(Number of bits), DAC/1(NOB)
  DAC/1(y) -> ZOH+comparator/2(DAC in), "           "/1
  ZOH+comparator/2(Output1) -> SAR/2(ZOH)
  SAR/1(Output) -> ZOH+comparator/3(Input)
  Trigger/1 -> ZOH+comparator/4(Clk), SAR/Trigger

== system MMADC/Sensing Channel 2/Sample&hold ==
  x(t) : Inport
  Trigger : Inport  Port=2
  Sample switch noise : Subsystem  TreatAsAtomicUnit=on
  Sample time jitter : Subsystem
  Sampled value : Outport
  wires:
  x(t)/1 -> Sample time jitter/1(x(t))
  Trigger/1 -> Sample switch noise/Trigger
  Sample switch noise/1(y(t)) -> Sampled value/1  "Sampled value"
  Sample time jitter/1(Output) -> Sample switch noise/1(Input)

== system MMADC/Sensing Channel 2/Subsystem2 ==
  Reset : Inport
  In1 : Inport  Port=2
  Trigger : TriggerPort  VariantControl=Variant  PortDimensions=1
  Add : Sum  Inputs=+++
  Multiply1 : Gain  Gain=MM_incomplete_transfer_coeff
  Multiply2 : Gain  Gain=MM_leakage_per_clk_cycle
  Random Number : RandomNumber  Variance=MM_sampling_noise  Seed=sim_number
  Subsystem : Subsystem
  Unit Delay : UnitDelay  SampleTime=-1  HasFrameUpgradeWarning=on
  Out1 : Outport
  wires:
  Add/1 -> Out1/1, Unit Delay/1
  Reset/1 -> Subsystem/1(In1)
  Subsystem/1(Out1) -> Add/3
  In1/1 -> Multiply1/1
  Unit Delay/1 -> Multiply2/1
  Multiply2/1 -> Subsystem/2(In2)
  Random Number/1 -> Add/1
  Multiply1/1 -> Add/2
